simulink model "ros"  (R2019a)
settings: Solver=VariableStepAuto  StartTime=0.0  StopTime=inf  RelTol=1e-3
libraries: robotlib x3
settings Model: Creator=24249  LastModifiedBy=huic

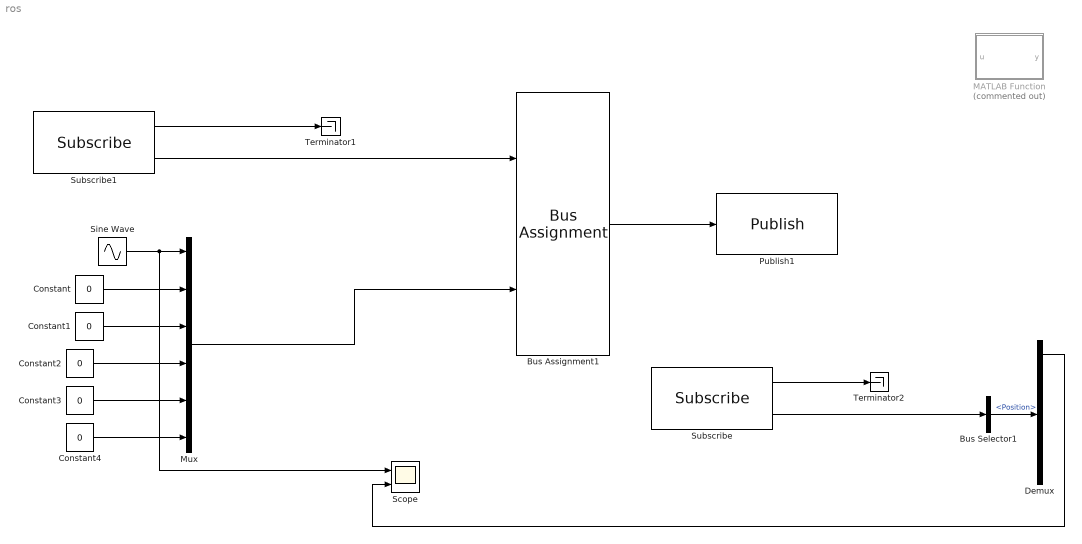
== system ros ==
  Bus Assignment1 : BusAssignment  AssignedSignals=Position
  Bus Selector1 : BusSelector  OutputSignals=Position
  Constant{,1..4} (5 alike) : Constant  Value=0
  Demux : Demux  Outputs=6
  MATLAB Function : MATLAB Function  Commented=on  TreatAsAtomicUnit=on
  Mux : Mux  Inputs=6
  Publish1 : robotlib/Publish  topicSource=Select from ROS network  topic=/joint_states  messageType=sensor_msgs/JointState  messageQueueLength=1
      settings: SourceProductBaseCode=RO
  Scope : Scope  NumInputPorts=2
  Sine Wave : Sin  SampleTime=0
  Subscribe : robotlib/Subscribe  topicSource=Select from ROS network  topic=/joint_states  messageType=sensor_msgs/JointState  sampleTime=-1  messageQueueLength=1
      settings: SourceProductBaseCode=RO
  Subscribe1 : robotlib/Subscribe  topicSource=Select from ROS network  topic=/myjoint_states  messageType=sensor_msgs/JointState  sampleTime=-1  messageQueueLength=1
      settings: SourceProductBaseCode=RO
  Terminator1 : Terminator
  Terminator2 : Terminator
  wires:
  Subscribe1/1 -> Terminator1/1
  Subscribe1/2 -> Bus Assignment1/1
  Bus Assignment1/1 -> Publish1/1
  Subscribe/1 -> Terminator2/1
  Subscribe/2 -> Bus Selector1/1
  Bus Selector1/1 -> Demux/1  "<Position>"
  Constant/1 -> Mux/2
  Constant1/1 -> Mux/3
  Constant2/1 -> Mux/4
  Constant3/1 -> Mux/5
  Constant4/1 -> Mux/6
  Mux/1 -> Bus Assignment1/2
  Demux/1 -> Scope/2
  Sine Wave/1 -> Scope/1, Mux/1

== matlab function ros/MATLAB Function ==
  data: u input; y output
function y = fcn(u)
%关节空间映射
y=zeros(1,6);
y(1) = 2.49*u(1);
y(2) = 1.794*u(2) + 1.57;
y(3) = 2.37*u(3) - 0.521;
y(4) = u(4) - 0.09;
y(5) = 2.169*u(5) - 1.355;
y(6) = 1.198*u(6);
